simulink model "switching_strategies_equivalences"  (Simulink 7.3)
settings: Solver=FixedStepDiscrete  StartTime=0.0  StopTime=10.0  FixedStep=0.02  RelTol=1e-3
libraries: voderiv x12
settings Model: Creator=Dominik  LastModifiedBy=dominik

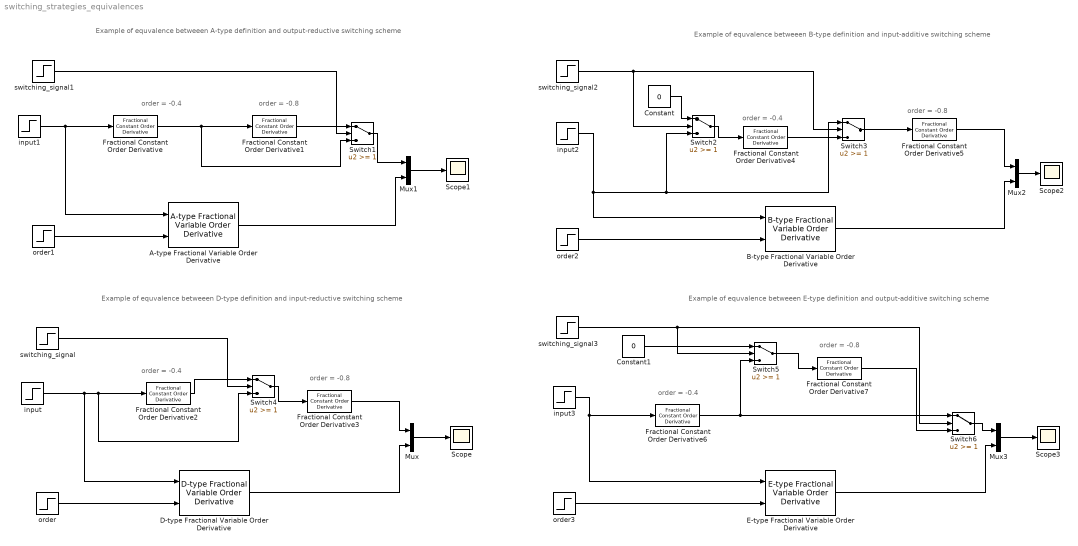
== system switching_strategies_equivalences ==
  note: Example of equvalence betweeen D-type definition
      |  and input-reductive switching scheme
  note: Example of equvalence betweeen A-type definition
      |  and output-reductive switching scheme
  note: Example of equvalence betweeen B-type definition
      |  and input-additive switching scheme
  note: Example of equvalence betweeen E-type definition
      |  and output-additive switching scheme
  note: order = -0.4
  note: order = -0.8
  note: order = -0.4
  note: order = -0.8
  note: order = -0.4
  note: order = -0.8
  note: order = -0.4
  note: order = -0.8
  A-type Fractional Variable Order Derivative : voderiv/A-type Fractional Variable Order Derivative  N=1  Nbuf=500  Ts=0.02
  B-type Fractional Variable Order Derivative : voderiv/B-type Fractional Variable Order Derivative  N=1  Nbuf=500  Ts=0.02
  Constant : Constant  Value=0  OutDataType=fixdt(1, 16)  OutScaling=2^0
  Constant1 : Constant  Value=0  OutDataType=fixdt(1, 16)  OutScaling=2^0
  D-type Fractional Variable Order Derivative : voderiv/D-type Fractional Variable Order Derivative  N=1  Nbuf=500  Ts=0.02
  E-type Fractional Variable Order Derivative : voderiv/E-type Fractional Variable Order Derivative  N=1  Nbuf=500  Ts=0.02
  Fractional Constant Order Derivative{,2,4,6} (4 alike) : voderiv/Fractional Constant Order Derivative  N=-0.4  Nbuf=500  Ts=0.02
  Fractional Constant Order Derivative{1,3,5,7} (4 alike) : voderiv/Fractional Constant Order Derivative  N=-0.8  Nbuf=500  Ts=0.02
  Mux{,1..3} (4 alike) : Mux  Inputs=2
  Scope{,1..3} (4 alike) : Scope
      Scope2 settings: SaveName=ScopeData2
      Scope3 settings: SaveName=ScopeData3
  Switch{1..6} (6 alike) : Switch  Threshold=1  OutDataType=fixdt(1, 16)  OutScaling=2^0
  input{,1..3} (4 alike) : Step  Time=0.5  SampleTime=0.02
  order : Step  Time=5  Before=-0.4-0.8  After=-0.8  SampleTime=0.02
  order1 : Step  Time=5  Before=-0.4-0.8  After=-0.4  SampleTime=0.02
  order2 : Step  Time=5  Before=-0.8  After=-0.4-0.8  SampleTime=0.02
  order3 : Step  Time=5  Before=-0.4  After=-0.4-0.8  SampleTime=0.02
  switching_signal{,1..3} (4 alike) : Step  Time=5  Before=1  After=0  SampleTime=0.02
  wires:
  input/1 -> Switch4/3, Fractional Constant Order Derivative2/1, D-type Fractional Variable Order Derivative/1
  Fractional Constant Order Derivative2/1 -> Switch4/1
  Switch4/1 -> Fractional Constant Order Derivative3/1
  Fractional Constant Order Derivative3/1 -> Mux/1
  Mux/1 -> Scope/1
  order/1 -> D-type Fractional Variable Order Derivative/2
  D-type Fractional Variable Order Derivative/1 -> Mux/2
  input1/1 -> Fractional Constant Order Derivative/1, A-type Fractional Variable Order Derivative/1
  Mux1/1 -> Scope1/1
  order1/1 -> A-type Fractional Variable Order Derivative/2
  A-type Fractional Variable Order Derivative/1 -> Mux1/2
  Fractional Constant Order Derivative/1 -> Switch1/3, Fractional Constant Order Derivative1/1
  Fractional Constant Order Derivative1/1 -> Switch1/1
  Switch1/1 -> Mux1/1
  switching_signal1/1 -> Switch1/2
  input2/1 -> Switch3/1, Switch2/3, B-type Fractional Variable Order Derivative/1
  Mux2/1 -> Scope2/1
  order2/1 -> B-type Fractional Variable Order Derivative/2
  B-type Fractional Variable Order Derivative/1 -> Mux2/2
  switching_signal2/1 -> Switch3/2, Switch2/2
  Switch3/1 -> Fractional Constant Order Derivative5/1
  Switch2/1 -> Fractional Constant Order Derivative4/1
  Constant/1 -> Switch2/1
  Fractional Constant Order Derivative4/1 -> Switch3/3
  Fractional Constant Order Derivative5/1 -> Mux2/1
  input3/1 -> Fractional Constant Order Derivative6/1, E-type Fractional Variable Order Derivative/1
  Mux3/1 -> Scope3/1
  order3/1 -> E-type Fractional Variable Order Derivative/2
  E-type Fractional Variable Order Derivative/1 -> Mux3/2
  switching_signal3/1 -> Switch5/2, Switch6/2
  Switch6/1 -> Mux3/1
  Fractional Constant Order Derivative6/1 -> Switch6/1, Switch5/3
  Fractional Constant Order Derivative7/1 -> Switch6/3
  Switch5/1 -> Fractional Constant Order Derivative7/1
  Constant1/1 -> Switch5/1
  switching_signal/1 -> Switch4/2
